simulink model "serial_vector_to_frdm"  (R2016b)
settings: Solver=FixedStepAuto  StartTime=0.0  StopTime=inf  RelTol=1e-3  EnableMultiTasking=on
libraries: simulink x3
settings Model: ExtModeTrigDuration=5  Creator=abz  LastModifiedBy=abz
settings OptimizationCC: MaxStackSize=64
settings DebuggingCC: ParameterTunabilityLossMsg=error
settings HardwareCC: ProdBitPerPointer=32  ProdBitPerSizeT=32  ProdBitPerPtrDiffT=32  ProdLargestAtomicInteger=Long  ProdLargestAtomicFloat=Double  ProdWordSize=32  ProdHWDeviceType=ARM Compatible->ARM Cortex
settings RTWCC: SystemTargetFile=ert.tlc  HardwareBoard=NXP FRDM-KL25Z  TLCOptions=-aInlineSetEventsForThisBaseRateFcn=TLC_FALSE -aSuppressMultiTaskScheduler=TLC_FALSE -aRateBasedStepFcn=1  TemplateMakefile=ert_default_tmf  Description=Embedded Coder  GenerateReport=on  Toolchain=GNU Tools for ARM Embedded Processors  IncludeHyperlinkInReport=on  LaunchReport=on  GenerateTraceInfo=on  GenerateTraceReport=on  GenerateTraceReportSl=on  GenerateTraceReportSf=on  GenerateTraceReportEml=on
settings CodeAppCC: ForceParamTrailComments=on  IgnoreCustomStorageClasses=off  OperatorAnnotations=on  SimulinkDataObjDesc=on  SFDataObjDesc=on  MATLABFcnDesc=on  InsertBlockDesc=on  MATLABSourceComments=on

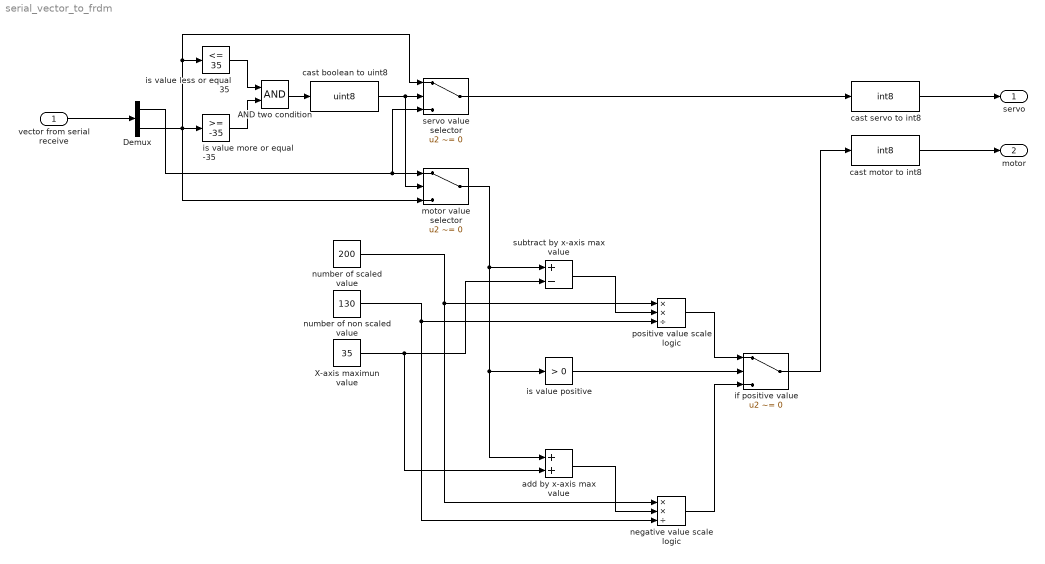
== system serial_vector_to_frdm ==
  vector from serial receive : Inport  OutDataTypeStr=int8
  AND two condition : Logic  AllPortsSameDT=off  OutDataTypeStr=boolean
  Demux : Demux  Outputs=2
  X-axis maximun value : Constant  Value=35
  add by x-axis max value : Sum
  cast boolean to uint8 : DataTypeConversion  OutDataTypeStr=uint8
  cast motor to int8 : DataTypeConversion  OutDataTypeStr=int8
  cast servo to int8 : DataTypeConversion  OutDataTypeStr=int8
  if positive value : Switch  Criteria=u2 ~= 0
  is value positive : simulink/Logic and Bit Operations/Compare To Constant  relop=>  const=0  OutDataTypeStr=uint8
  is value less or equal 35 : simulink/Logic and Bit Operations/Compare To Constant  relop=<=  const=35  OutDataTypeStr=boolean
  is value more or equal -35 : simulink/Logic and Bit Operations/Compare To Constant  relop=>=  const=-35  OutDataTypeStr=boolean
  "motor value selector " : Switch  Criteria=u2 ~= 0
  negative value scale logic : Product  Inputs=**/
  number of non scaled value : Constant  Value=130
  number of scaled value : Constant  Value=200
  positive value scale logic : Product  Inputs=**/
  servo value selector : Switch  Criteria=u2 ~= 0
  subtract by x-axis max value : Sum  Inputs=+-
  servo : Outport
  motor : Outport  Port=2
  wires:
  servo value selector/1 -> cast servo to int8/1
  is value less or equal 35/1 -> AND two condition/1
  is value more or equal -35/1 -> AND two condition/2
  Demux/2 -> is value less or equal 35/1, servo value selector/1, is value more or equal -35/1, "motor value selector "/3
  Demux/1 -> "motor value selector "/1, servo value selector/3
  cast boolean to uint8/1 -> servo value selector/2, "motor value selector "/2
  is value positive/1 -> if positive value/2
  "motor value selector "/1 -> subtract by x-axis max value/1, add by x-axis max value/1, is value positive/1
  vector from serial receive/1 -> Demux/1
  if positive value/1 -> cast motor to int8/1
  AND two condition/1 -> cast boolean to uint8/1
  cast servo to int8/1 -> servo/1
  cast motor to int8/1 -> motor/1
  number of scaled value/1 -> negative value scale logic/1, positive value scale logic/1
  number of non scaled value/1 -> negative value scale logic/3, positive value scale logic/3
  X-axis maximun value/1 -> subtract by x-axis max value/2, add by x-axis max value/2
  add by x-axis max value/1 -> negative value scale logic/2
  subtract by x-axis max value/1 -> positive value scale logic/2
  positive value scale logic/1 -> if positive value/1
  negative value scale logic/1 -> if positive value/3
